simulink subsystem "SensoresAj"  (R2023b)
settings: Solver=VariableStepAuto  StartTime=0.0  StopTime=10.0  RelTol=1e-3
libraries: arduinolib x2
settings Model: Creator=USUARIO  LastModifiedBy=USUARIO

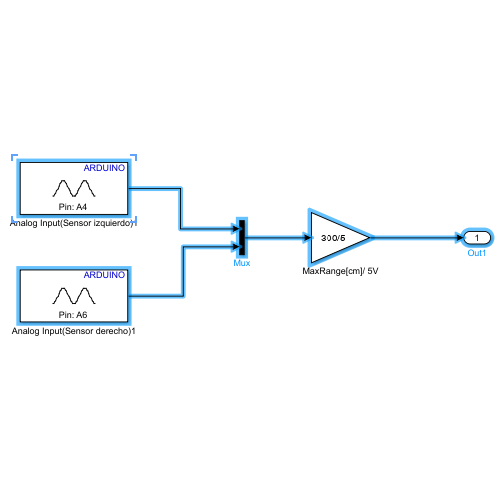
[thumbnail: Simulink's stored preview of the top-level diagram]
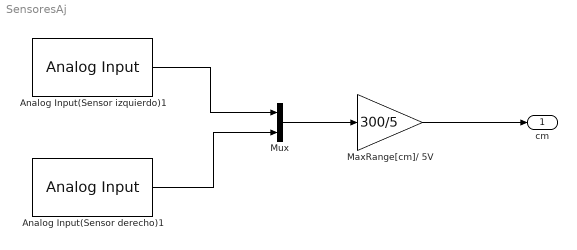
== system SensoresAj ==
  Analog Input(Sensor derecho)1 : arduinolib/Analog Input  pinNumber=6  ReadResultsOnly=off  ConversionTriggerSource=Software  ExternalTriggerType=uint32( 0 )  OutputDataType=uint16  EnableConversionCompleteNotify=off  EnableOuputStatus=off  SampleTime=0.01  blockPlatform=arduino
  Analog Input(Sensor izquierdo)1 : arduinolib/Analog Input  pinNumber=4  ReadResultsOnly=off  ConversionTriggerSource=Software  ExternalTriggerType=uint32( 0 )  OutputDataType=uint16  EnableConversionCompleteNotify=off  EnableOuputStatus=off  SampleTime=0.01  blockPlatform=arduino
  MaxRange[cm]/ 5V : Gain  Gain=300/5  OutDataTypeStr=double
  Mux : Mux  Inputs=2
  cm : Outport
  wires:
  MaxRange[cm]/ 5V/1 -> cm/1
  Analog Input(Sensor izquierdo)1/1 -> Mux/1
  Mux/1 -> MaxRange[cm]/ 5V/1
  Analog Input(Sensor derecho)1/1 -> Mux/2
